simulink model "manul_model_stage15_complete_pre_engineering_20260816"  (R2025a)
settings: Solver=ode3  StartTime=0.0  StopTime=0.3  FixedStep=Ts_power  RelTol=1e-3
InitFcn:
  | run('D:/PV_MPPT/PV_ESS_MPC_Manul_Reproduction/experiments/stage15_bus_stability_20260814/pvess_stage15_busfix_init.m')
values from neighbouring files (symbols this model uses):
  Ad_mpvc = expm(A_mpvc*Ts_mpc)    [pvess_beginner_init_baseline.m]    (also in pvess_stage15_busfix_init.m; pvess_stage15_busfix_init_pre_cpl_20260817.m; pvess_stage15_busfix_init_pre_engineering_20260816.m; pvess_stage15_busfix_init_pre_gridpi_tuning_20260817.m)
  Bd_mpvc = A_mpvc\((Ad_mpvc-eye(2))*B_mpvc)    [pvess_beginner_init_baseline.m]    (also in pvess_stage15_busfix_init.m; pvess_stage15_busfix_init_pre_cpl_20260817.m; pvess_stage15_busfix_init_pre_engineering_20260816.m; pvess_stage15_busfix_init_pre_gridpi_tuning_20260817.m)
  Cdc = 18e-3    (= 0.018)    [pvess_beginner_init_baseline.m]    (also in pvess_stage15_busfix_init.m; pvess_stage15_busfix_init_pre_cpl_20260817.m; pvess_stage15_busfix_init_pre_engineering_20260816.m; pvess_stage15_busfix_init_pre_gridpi_tuning_20260817.m)
  Cpv = 10e-3    (= 0.01)    [pvess_beginner_init_baseline.m]    (also in pvess_stage15_busfix_init.m; pvess_stage15_busfix_init_pre_cpl_20260817.m; pvess_stage15_busfix_init_pre_engineering_20260816.m; pvess_stage15_busfix_init_pre_gridpi_tuning_20260817.m)
  Db0 = 1 - V_bat_nom/Vdc_ref    (= 0.75)    [pvess_beginner_init_baseline.m]    (also in pvess_stage15_busfix_init.m; pvess_stage15_busfix_init_pre_cpl_20260817.m; pvess_stage15_busfix_init_pre_engineering_20260816.m; pvess_stage15_busfix_init_pre_gridpi_tuning_20260817.m)
  Db_max = 0.95    [pvess_beginner_init_baseline.m]    (also in pvess_stage15_busfix_init.m; pvess_stage15_busfix_init_pre_cpl_20260817.m; pvess_stage15_busfix_init_pre_engineering_20260816.m; pvess_stage15_busfix_init_pre_gridpi_tuning_20260817.m)
  Db_min = 0.05    [pvess_beginner_init_baseline.m]    (also in pvess_stage15_busfix_init.m; pvess_stage15_busfix_init_pre_cpl_20260817.m; pvess_stage15_busfix_init_pre_engineering_20260816.m; pvess_stage15_busfix_init_pre_gridpi_tuning_20260817.m)
  Dpv0 = 1 - 547/Vdc_ref    (= 0.544166666667)    [pvess_beginner_init_baseline.m]    (also in pvess_stage15_busfix_init.m; pvess_stage15_busfix_init_pre_cpl_20260817.m; pvess_stage15_busfix_init_pre_engineering_20260816.m; pvess_stage15_busfix_init_pre_gridpi_tuning_20260817.m)
  Dpv_curtail_bias = 0.506    [pvess_stage15_busfix_init.m]    (also in pvess_stage15_busfix_init_pre_cpl_20260817.m; pvess_stage15_busfix_init_pre_engineering_20260816.m; pvess_stage15_busfix_init_pre_gridpi_tuning_20260817.m)
  Dpv_max = 0.75    [pvess_beginner_init_baseline.m]    (also in pvess_stage15_busfix_init.m; pvess_stage15_busfix_init_pre_cpl_20260817.m; pvess_stage15_busfix_init_pre_engineering_20260816.m; pvess_stage15_busfix_init_pre_gridpi_tuning_20260817.m)
  Dpv_min = 0.35    [pvess_beginner_init_baseline.m]    (also in pvess_stage15_busfix_init.m; pvess_stage15_busfix_init_pre_cpl_20260817.m; pvess_stage15_busfix_init_pre_engineering_20260816.m; pvess_stage15_busfix_init_pre_gridpi_tuning_20260817.m)
  Dpv_slew_down = -5.0    (= -5)    [pvess_stage15_busfix_init.m]    (also in pvess_stage15_busfix_init_pre_cpl_20260817.m; pvess_stage15_busfix_init_pre_engineering_20260816.m; pvess_stage15_busfix_init_pre_gridpi_tuning_20260817.m)
  Dpv_slew_up = 1.0    (= 1)    [pvess_stage15_busfix_init.m]    (also in pvess_stage15_busfix_init_pre_cpl_20260817.m; pvess_stage15_busfix_init_pre_engineering_20260816.m; pvess_stage15_busfix_init_pre_gridpi_tuning_20260817.m)
  Dpv_step = 2e-4    (= 0.0002)    [pvess_beginner_init_baseline.m]    (also in pvess_stage15_busfix_init.m; pvess_stage15_busfix_init_pre_cpl_20260817.m; pvess_stage15_busfix_init_pre_engineering_20260816.m; pvess_stage15_busfix_init_pre_gridpi_tuning_20260817.m)
  eps_dI = 1e-3    (= 0.001)    [pvess_beginner_init_baseline.m]    (also in pvess_stage15_busfix_init.m; pvess_stage15_busfix_init_pre_cpl_20260817.m; pvess_stage15_busfix_init_pre_engineering_20260816.m; pvess_stage15_busfix_init_pre_gridpi_tuning_20260817.m)
  eps_dV = 1e-3    (= 0.001)    [pvess_beginner_init_baseline.m]    (also in pvess_stage15_busfix_init.m; pvess_stage15_busfix_init_pre_cpl_20260817.m; pvess_stage15_busfix_init_pre_engineering_20260816.m; pvess_stage15_busfix_init_pre_gridpi_tuning_20260817.m)
  eps_inc = 1e-4    (= 0.0001)    [pvess_beginner_init_baseline.m]    (also in pvess_stage15_busfix_init.m; pvess_stage15_busfix_init_pre_cpl_20260817.m; pvess_stage15_busfix_init_pre_engineering_20260816.m; pvess_stage15_busfix_init_pre_gridpi_tuning_20260817.m)
  f_grid = 50    [pvess_beginner_init_baseline.m]    (also in pvess_stage15_busfix_init.m; pvess_stage15_busfix_init_pre_cpl_20260817.m; pvess_stage15_busfix_init_pre_engineering_20260816.m; pvess_stage15_busfix_init_pre_gridpi_tuning_20260817.m)
  freq_threshold = 0.15    [pvess_beginner_init_baseline.m]    (also in pvess_stage15_busfix_init.m; pvess_stage15_busfix_init_pre_cpl_20260817.m; pvess_stage15_busfix_init_pre_engineering_20260816.m; pvess_stage15_busfix_init_pre_gridpi_tuning_20260817.m)
  Ibat_curtail_release = -0.8*Ibat_max    (= -1333.33333333)    [pvess_stage15_busfix_init.m]    (also in pvess_stage15_busfix_init_pre_cpl_20260817.m; pvess_stage15_busfix_init_pre_engineering_20260816.m; pvess_stage15_busfix_init_pre_gridpi_tuning_20260817.m)
  Ibat_max = P_bat_rated/V_bat_nom    (= 1666.66666667)    [pvess_beginner_init_baseline.m]    (also in pvess_stage15_busfix_init.m; pvess_stage15_busfix_init_pre_cpl_20260817.m; pvess_stage15_busfix_init_pre_engineering_20260816.m; pvess_stage15_busfix_init_pre_gridpi_tuning_20260817.m)
  K_bat_sign = 1    [pvess_beginner_init_baseline.m]    (also in pvess_stage15_busfix_init.m; pvess_stage15_busfix_init_pre_cpl_20260817.m; pvess_stage15_busfix_init_pre_engineering_20260816.m; pvess_stage15_busfix_init_pre_gridpi_tuning_20260817.m)
  K_grid_sign = -1    [pvess_beginner_init_baseline.m]    (also in pvess_stage15_busfix_init.m; pvess_stage15_busfix_init_pre_cpl_20260817.m; pvess_stage15_busfix_init_pre_engineering_20260816.m; pvess_stage15_busfix_init_pre_gridpi_tuning_20260817.m)
  Ki_dc = 3.40748e5    (= 340748)    [pvess_beginner_init_baseline.m]    (also in pvess_stage15_busfix_init.m = 2131834.55064; pvess_stage15_busfix_init_pre_cpl_20260817.m; pvess_stage15_busfix_init_pre_engineering_20260816.m; pvess_stage15_busfix_init_pre_gridpi_tuning_20260817.m)
  Kii_bat = 0.150    (= 0.15)    [pvess_beginner_init_baseline.m]    (also in pvess_stage15_busfix_init.m = 0.05; pvess_stage15_busfix_init_pre_cpl_20260817.m = 0.05; pvess_stage15_busfix_init_pre_engineering_20260816.m = 0.05; pvess_stage15_busfix_init_pre_gridpi_tuning_20260817.m = 0.05)
  Kiv_bat = 650    [pvess_beginner_init_baseline.m]    (also in pvess_stage15_busfix_init.m; pvess_stage15_busfix_init_pre_cpl_20260817.m; pvess_stage15_busfix_init_pre_engineering_20260816.m; pvess_stage15_busfix_init_pre_gridpi_tuning_20260817.m)
  Kp_dc = 3836.125    [pvess_beginner_init_baseline.m]    (also in pvess_stage15_busfix_init.m = 2*zeta_dc*(2*pi*f_bw_dc)*Cdc*Vdc_ref; pvess_stage15_busfix_init_pre_cpl_20260817.m; pvess_stage15_busfix_init_pre_engineering_20260816.m; pvess_stage15_busfix_init_pre_gridpi_tuning_20260817.m)
  Kp_pv_curtail = 5e-5    (= 5e-05)    [pvess_stage15_busfix_init.m]    (also in pvess_stage15_busfix_init_pre_cpl_20260817.m; pvess_stage15_busfix_init_pre_engineering_20260816.m; pvess_stage15_busfix_init_pre_gridpi_tuning_20260817.m)
  Kpi_bat = 100e-3    (= 0.1)    [pvess_beginner_init_baseline.m]    (also in pvess_stage15_busfix_init.m = 0.005; pvess_stage15_busfix_init_pre_cpl_20260817.m = 0.005; pvess_stage15_busfix_init_pre_engineering_20260816.m = 0.005; pvess_stage15_busfix_init_pre_gridpi_tuning_20260817.m = 0.005)
  Kpv_bat = 4    [pvess_beginner_init_baseline.m]    (also in pvess_stage15_busfix_init.m; pvess_stage15_busfix_init_pre_cpl_20260817.m; pvess_stage15_busfix_init_pre_engineering_20260816.m; pvess_stage15_busfix_init_pre_gridpi_tuning_20260817.m)
  lambda_mppc = 0.001    [pvess_beginner_init_baseline.m]    (also in pvess_stage15_busfix_init.m; pvess_stage15_busfix_init_pre_cpl_20260817.m; pvess_stage15_busfix_init_pre_engineering_20260816.m; pvess_stage15_busfix_init_pre_gridpi_tuning_20260817.m)
  lambda_mpvc = 3e-6    (= 3e-06)    [pvess_beginner_init_baseline.m]    (also in pvess_stage15_busfix_init.m; pvess_stage15_busfix_init_pre_cpl_20260817.m; pvess_stage15_busfix_init_pre_engineering_20260816.m; pvess_stage15_busfix_init_pre_gridpi_tuning_20260817.m)
  Lbat = 11.25e-3    (= 0.01125)    [pvess_beginner_init_baseline.m]    (also in pvess_stage15_busfix_init.m = 0.0005; pvess_stage15_busfix_init_pre_cpl_20260817.m = 0.0005; pvess_stage15_busfix_init_pre_engineering_20260816.m = 0.0005; pvess_stage15_busfix_init_pre_gridpi_tuning_20260817.m = 0.0005)
  Lf = 0.6e-3    (= 0.0006)    [pvess_beginner_init_baseline.m]    (also in pvess_stage15_busfix_init.m; pvess_stage15_busfix_init_pre_cpl_20260817.m; pvess_stage15_busfix_init_pre_engineering_20260816.m; pvess_stage15_busfix_init_pre_gridpi_tuning_20260817.m)
  Lpv = 0.8e-3    (= 0.0008)    [pvess_beginner_init_baseline.m]    (also in pvess_stage15_busfix_init.m; pvess_stage15_busfix_init_pre_cpl_20260817.m; pvess_stage15_busfix_init_pre_engineering_20260816.m; pvess_stage15_busfix_init_pre_gridpi_tuning_20260817.m)
  m_var = 4e6    (= 4000000)    [pvess_beginner_init_baseline.m]    (also in pvess_stage15_busfix_init.m; pvess_stage15_busfix_init_pre_cpl_20260817.m; pvess_stage15_busfix_init_pre_engineering_20260816.m; pvess_stage15_busfix_init_pre_gridpi_tuning_20260817.m)
  N_ems_fast_avg = 100    [pvess_beginner_init_baseline.m]    (also in pvess_stage15_busfix_init.m; pvess_stage15_busfix_init_pre_cpl_20260817.m; pvess_stage15_busfix_init_pre_engineering_20260816.m; pvess_stage15_busfix_init_pre_gridpi_tuning_20260817.m)
  omega_grid = 2*pi*f_grid    (= 314.159265359)    [pvess_beginner_init_baseline.m]    (also in pvess_stage15_busfix_init.m; pvess_stage15_busfix_init_pre_cpl_20260817.m; pvess_stage15_busfix_init_pre_engineering_20260816.m; pvess_stage15_busfix_init_pre_gridpi_tuning_20260817.m)
  P_base_mpc = 2e6    (= 2000000)    [pvess_beginner_init_baseline.m]    (also in pvess_stage15_busfix_init.m; pvess_stage15_busfix_init_pre_cpl_20260817.m; pvess_stage15_busfix_init_pre_engineering_20260816.m; pvess_stage15_busfix_init_pre_gridpi_tuning_20260817.m)
  phase_threshold = 0.99863    [pvess_beginner_init_baseline.m]    (also in pvess_stage15_busfix_init.m; pvess_stage15_busfix_init_pre_cpl_20260817.m; pvess_stage15_busfix_init_pre_engineering_20260816.m; pvess_stage15_busfix_init_pre_gridpi_tuning_20260817.m)
  Pref_max = 2.2e6    (= 2200000)    [pvess_beginner_init_baseline.m]    (also in pvess_stage15_busfix_init.m; pvess_stage15_busfix_init_pre_cpl_20260817.m; pvess_stage15_busfix_init_pre_engineering_20260816.m; pvess_stage15_busfix_init_pre_gridpi_tuning_20260817.m)
  Pref_min = -2.2e6    (= -2200000)    [pvess_beginner_init_baseline.m]    (also in pvess_stage15_busfix_init.m; pvess_stage15_busfix_init_pre_cpl_20260817.m; pvess_stage15_busfix_init_pre_engineering_20260816.m; pvess_stage15_busfix_init_pre_gridpi_tuning_20260817.m)
  Q_base_mpc = 1e6    (= 1000000)    [pvess_beginner_init_baseline.m]    (also in pvess_stage15_busfix_init.m; pvess_stage15_busfix_init_pre_cpl_20260817.m; pvess_stage15_busfix_init_pre_engineering_20260816.m; pvess_stage15_busfix_init_pre_gridpi_tuning_20260817.m)
  Q_bat_Ah = 1300    [pvess_beginner_init_baseline.m]    (also in pvess_stage15_busfix_init.m; pvess_stage15_busfix_init_pre_cpl_20260817.m; pvess_stage15_busfix_init_pre_engineering_20260816.m; pvess_stage15_busfix_init_pre_gridpi_tuning_20260817.m)
  R_bat_internal = 0.02    [pvess_beginner_init_baseline.m]    (also in pvess_stage15_busfix_init.m; pvess_stage15_busfix_init_pre_cpl_20260817.m; pvess_stage15_busfix_init_pre_engineering_20260816.m; pvess_stage15_busfix_init_pre_gridpi_tuning_20260817.m)
  Rf = 0.019    [pvess_beginner_init_baseline.m]    (also in pvess_stage15_busfix_init.m; pvess_stage15_busfix_init_pre_cpl_20260817.m; pvess_stage15_busfix_init_pre_engineering_20260816.m; pvess_stage15_busfix_init_pre_gridpi_tuning_20260817.m)
  RLbat = 2e-3    (= 0.002)    [pvess_beginner_init_baseline.m]    (also in pvess_stage15_busfix_init.m; pvess_stage15_busfix_init_pre_cpl_20260817.m; pvess_stage15_busfix_init_pre_engineering_20260816.m; pvess_stage15_busfix_init_pre_gridpi_tuning_20260817.m)
  RLpv = 2e-3    (= 0.002)    [pvess_beginner_init_baseline.m]    (also in pvess_stage15_busfix_init.m; pvess_stage15_busfix_init_pre_cpl_20260817.m; pvess_stage15_busfix_init_pre_engineering_20260816.m; pvess_stage15_busfix_init_pre_gridpi_tuning_20260817.m)
  S_tr = 2.5e6    (= 2500000)    [pvess_beginner_init_baseline.m]    (also in pvess_stage15_busfix_init.m; pvess_stage15_busfix_init_pre_cpl_20260817.m; pvess_stage15_busfix_init_pre_engineering_20260816.m; pvess_stage15_busfix_init_pre_gridpi_tuning_20260817.m)
  SOC0 = 50    [pvess_beginner_init_baseline.m]    (also in pvess_stage15_busfix_init.m; pvess_stage15_busfix_init_pre_cpl_20260817.m; pvess_stage15_busfix_init_pre_engineering_20260816.m; pvess_stage15_busfix_init_pre_gridpi_tuning_20260817.m)
  SOC_max = 90    [pvess_beginner_init_baseline.m]    (also in pvess_stage15_busfix_init.m; pvess_stage15_busfix_init_pre_cpl_20260817.m; pvess_stage15_busfix_init_pre_engineering_20260816.m; pvess_stage15_busfix_init_pre_gridpi_tuning_20260817.m)
  SOC_min = 10    [pvess_beginner_init_baseline.m]    (also in pvess_stage15_busfix_init.m; pvess_stage15_busfix_init_pre_cpl_20260817.m; pvess_stage15_busfix_init_pre_engineering_20260816.m; pvess_stage15_busfix_init_pre_gridpi_tuning_20260817.m)
  sync_hold = 0.1    [pvess_beginner_init_baseline.m]    (also in pvess_stage15_busfix_init.m; pvess_stage15_busfix_init_pre_cpl_20260817.m; pvess_stage15_busfix_init_pre_engineering_20260816.m; pvess_stage15_busfix_init_pre_gridpi_tuning_20260817.m)
  T_ac_step = 0.2    [pvess_beginner_init_baseline.m]    (also in pvess_stage15_busfix_init.m = 0.5; pvess_stage15_busfix_init_pre_cpl_20260817.m = 0.5; pvess_stage15_busfix_init_pre_engineering_20260816.m = 0.5; pvess_stage15_busfix_init_pre_gridpi_tuning_20260817.m = 0.5)
  T_grid_connect = 1.6    [pvess_beginner_init_baseline.m]    (also in pvess_stage15_busfix_init.m; pvess_stage15_busfix_init_pre_cpl_20260817.m; pvess_stage15_busfix_init_pre_engineering_20260816.m; pvess_stage15_busfix_init_pre_gridpi_tuning_20260817.m)
  T_grid_dip = 3.5    [pvess_beginner_init_baseline.m]    (also in pvess_stage15_busfix_init.m; pvess_stage15_busfix_init_pre_cpl_20260817.m; pvess_stage15_busfix_init_pre_engineering_20260816.m; pvess_stage15_busfix_init_pre_gridpi_tuning_20260817.m)
  T_sync = 1.4    [pvess_beginner_init_baseline.m]    (also in pvess_stage15_busfix_init.m; pvess_stage15_busfix_init_pre_cpl_20260817.m; pvess_stage15_busfix_init_pre_engineering_20260816.m; pvess_stage15_busfix_init_pre_gridpi_tuning_20260817.m)
  Ts_bat_ctrl = 100e-6    (= 0.0001)    [pvess_beginner_init_baseline.m]    (also in pvess_stage15_busfix_init.m; pvess_stage15_busfix_init_pre_cpl_20260817.m; pvess_stage15_busfix_init_pre_engineering_20260816.m; pvess_stage15_busfix_init_pre_gridpi_tuning_20260817.m)
  Ts_ems = 1e-3    (= 0.001)    [pvess_beginner_init_baseline.m]    (also in pvess_stage15_busfix_init.m; pvess_stage15_busfix_init_pre_cpl_20260817.m; pvess_stage15_busfix_init_pre_engineering_20260816.m; pvess_stage15_busfix_init_pre_gridpi_tuning_20260817.m)
  Ts_mpc = 1/20e3    (= 5e-05)    [pvess_beginner_init_baseline.m]    (also in pvess_stage15_busfix_init.m; pvess_stage15_busfix_init_pre_cpl_20260817.m; pvess_stage15_busfix_init_pre_engineering_20260816.m; pvess_stage15_busfix_init_pre_gridpi_tuning_20260817.m)
  Ts_mppt = 1e-3    (= 0.001)    [pvess_beginner_init_baseline.m]    (also in pvess_stage15_busfix_init.m; pvess_stage15_busfix_init_pre_cpl_20260817.m; pvess_stage15_busfix_init_pre_engineering_20260816.m; pvess_stage15_busfix_init_pre_gridpi_tuning_20260817.m)
  Ts_power = 2e-6    (= 2e-06)    [pvess_beginner_init_baseline.m]    (also in pvess_stage15_busfix_init.m; pvess_stage15_busfix_init_pre_cpl_20260817.m; pvess_stage15_busfix_init_pre_engineering_20260816.m; pvess_stage15_busfix_init_pre_gridpi_tuning_20260817.m)
  Ts_soc = 1e-4    (= 0.0001)    [pvess_beginner_init_baseline.m]    (also in pvess_stage15_busfix_init.m; pvess_stage15_busfix_init_pre_cpl_20260817.m; pvess_stage15_busfix_init_pre_engineering_20260816.m; pvess_stage15_busfix_init_pre_gridpi_tuning_20260817.m)
  V_bat_nom = 300    [pvess_beginner_init_baseline.m]    (also in pvess_stage15_busfix_init.m; pvess_stage15_busfix_init_pre_cpl_20260817.m; pvess_stage15_busfix_init_pre_engineering_20260816.m; pvess_stage15_busfix_init_pre_gridpi_tuning_20260817.m)
  V_tr_hv = 25e3    (= 25000)    [pvess_beginner_init_baseline.m]    (also in pvess_stage15_busfix_init.m; pvess_stage15_busfix_init_pre_cpl_20260817.m; pvess_stage15_busfix_init_pre_engineering_20260816.m; pvess_stage15_busfix_init_pre_gridpi_tuning_20260817.m)
  V_tr_lv = Vac_ll    (= 690)    [pvess_beginner_init_baseline.m]    (also in pvess_stage15_busfix_init.m; pvess_stage15_busfix_init_pre_cpl_20260817.m; pvess_stage15_busfix_init_pre_engineering_20260816.m; pvess_stage15_busfix_init_pre_gridpi_tuning_20260817.m)
  Vac_phase_peak = sqrt(2)*Vac_ll/sqrt(3)    [pvess_beginner_init_baseline.m]    (also in pvess_stage15_busfix_init.m; pvess_stage15_busfix_init_pre_cpl_20260817.m; pvess_stage15_busfix_init_pre_engineering_20260816.m; pvess_stage15_busfix_init_pre_gridpi_tuning_20260817.m)
  Vdc_curtail_off = 1185    [pvess_stage15_busfix_init.m]    (also in pvess_stage15_busfix_init_pre_cpl_20260817.m; pvess_stage15_busfix_init_pre_engineering_20260816.m; pvess_stage15_busfix_init_pre_gridpi_tuning_20260817.m)
  Vdc_curtail_on = 1220    [pvess_stage15_busfix_init.m]    (also in pvess_stage15_busfix_init_pre_cpl_20260817.m; pvess_stage15_busfix_init_pre_engineering_20260816.m; pvess_stage15_busfix_init_pre_gridpi_tuning_20260817.m)
  Vdc_ref = 1200    [pvess_beginner_init_baseline.m]    (also in pvess_stage15_busfix_init.m; pvess_stage15_busfix_init_pre_cpl_20260817.m; pvess_stage15_busfix_init_pre_engineering_20260816.m; pvess_stage15_busfix_init_pre_gridpi_tuning_20260817.m)
  Vf_diode = 1.0    (= 1)    [pvess_beginner_init_baseline.m]    (also in pvess_stage15_busfix_init.m; pvess_stage15_busfix_init_pre_cpl_20260817.m; pvess_stage15_busfix_init_pre_engineering_20260816.m; pvess_stage15_busfix_init_pre_gridpi_tuning_20260817.m)
  Vpv0 = 547    [pvess_beginner_init_baseline.m]    (also in pvess_stage15_busfix_init.m; pvess_stage15_busfix_init_pre_cpl_20260817.m; pvess_stage15_busfix_init_pre_engineering_20260816.m; pvess_stage15_busfix_init_pre_gridpi_tuning_20260817.m)
  Vsync_threshold = 10    [pvess_beginner_init_baseline.m]    (also in pvess_stage15_busfix_init.m; pvess_stage15_busfix_init_pre_cpl_20260817.m; pvess_stage15_busfix_init_pre_engineering_20260816.m; pvess_stage15_busfix_init_pre_gridpi_tuning_20260817.m)
undefined symbols (not defined in the file or in its folder): DiscIntNeverNeededParam, dspblkCoreblockFVToolHelper, gcbh, Ion, Kt_dc, Lithium
libraries: dspstat3 x10, simulink x9, spsBreakerLib x5, spsCurrentMeasurementLib x4, slpidlib x3, spsThreePhaseVIMeasurementLib x3, eeRmsMeasurement x3, spsThreePhaseParallelRLCLoadLib x3, spsThreePhaseBreakerLib x3, spsParallelRLCBranchLib x2, spsVariableResistorLib x2, spsThreePhaseSeriesRLCBranchLib x2
(part 2 of 2)

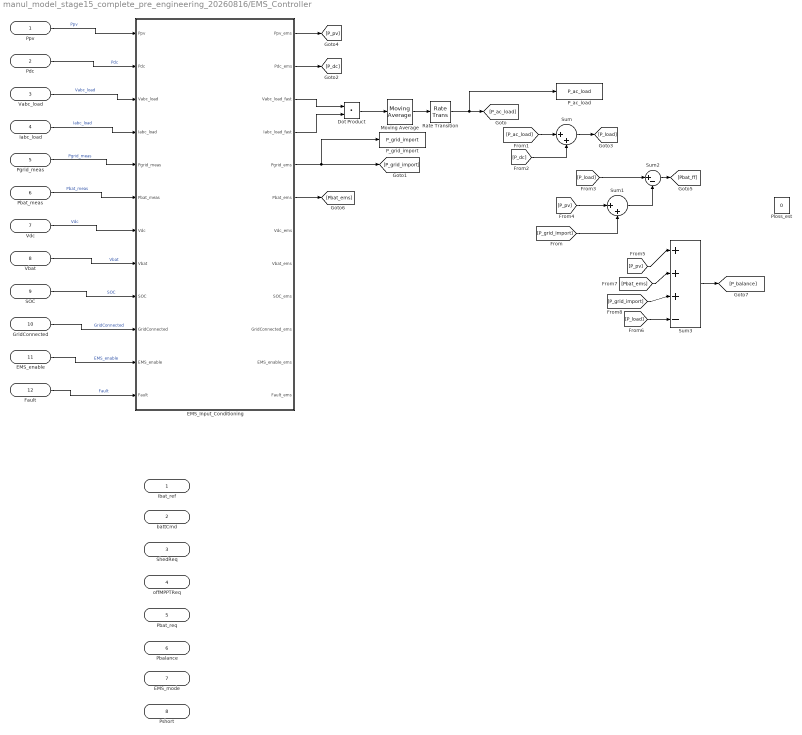
== system manul_model_stage15_complete_pre_engineering_20260816/EMS_Controller ==
  Ppv : Inport  OutDataTypeStr=double  PortDimensions=1  SampleTime=Ts_power
  Pdc : Inport  Port=2  OutDataTypeStr=double  PortDimensions=1  SampleTime=Ts_power
  Vabc_load : Inport  Port=3  OutDataTypeStr=double  PortDimensions=3  SampleTime=Ts_mpc
  Iabc_load : Inport  Port=4  OutDataTypeStr=double  PortDimensions=3  SampleTime=Ts_mpc
  Pgrid_meas : Inport  Port=5  OutDataTypeStr=double  PortDimensions=1  SampleTime=Ts_mpc
  Pbat_meas : Inport  Port=6  OutDataTypeStr=double  PortDimensions=1  SampleTime=Ts_power
  Vdc : Inport  Port=7  OutDataTypeStr=double  PortDimensions=1  SampleTime=Ts_power
  Vbat : Inport  Port=8  OutDataTypeStr=double  PortDimensions=1  SampleTime=Ts_power
  SOC : Inport  Port=9  OutDataTypeStr=double  PortDimensions=1  SampleTime=Ts_soc
  GridConnected : Inport  Port=10  OutDataTypeStr=boolean  PortDimensions=1
  EMS_enable : Inport  Port=11  OutDataTypeStr=boolean  PortDimensions=1
  Fault : Inport  Port=12  OutDataTypeStr=boolean  PortDimensions=1
  Dot Product : DotProduct  OutDataTypeStr=Inherit: Inherit via internal rule
  EMS_Input_Conditioning : Subsystem
  Moving Average : dspstat3/Moving Average  Method=Sliding window  ForgettingFactorPort=off  SpecifyWindowLength=on  WindowLength=20  OverlapLength=19  AllowArbitraryInputLength=off  ForgettingFactor=0.9  SimulateUsing=Interpreted execution
  P_ac_load : ToWorkspace  VariableName=P_ac_load  SaveFormat=Timeseries  SampleTime=-1
  P_grid_import : ToWorkspace  VariableName=P_grid_import  SaveFormat=Timeseries  SampleTime=-1
  Ploss_est : Constant  Value=0
  Rate Transition : RateTransition  OutPortSampleTime=Ts_ems
  Sum : Sum  Inputs=|++
  Sum1 : Sum  Inputs=|++
  Sum2 : Sum  Inputs=|+-
  Sum3 : Sum  Inputs=|+++-
  Ibat_ref : Outport  OutDataTypeStr=double  PortDimensions=1
  battCmd : Outport  Port=2  OutDataTypeStr=int8  PortDimensions=1
  ShedReq : Outport  Port=3  OutDataTypeStr=boolean  PortDimensions=1
  offMPPTReq : Outport  Port=4  OutDataTypeStr=boolean  PortDimensions=1
  Pbat_req : Outport  Port=5  OutDataTypeStr=double  PortDimensions=1
  Pbalance : Outport  Port=6  OutDataTypeStr=double  PortDimensions=1
  EMS_mode : Outport  Port=7  OutDataTypeStr=int8  PortDimensions=1
  Pshort : Outport  Port=8  OutDataTypeStr=double  PortDimensions=1
  wires:
  Ppv/1 -> EMS_Input_Conditioning/1(Ppv)  "Ppv"
  Pdc/1 -> EMS_Input_Conditioning/2(Pdc)  "Pdc"
  Vabc_load/1 -> EMS_Input_Conditioning/3(Vabc_load)  "Vabc_load"
  Iabc_load/1 -> EMS_Input_Conditioning/4(Iabc_load)  "Iabc_load"
  Pgrid_meas/1 -> EMS_Input_Conditioning/5(Pgrid_meas)  "Pgrid_meas"
  Pbat_meas/1 -> EMS_Input_Conditioning/6(Pbat_meas)  "Pbat_meas"
  Vdc/1 -> EMS_Input_Conditioning/7(Vdc)  "Vdc"
  Vbat/1 -> EMS_Input_Conditioning/8(Vbat)  "Vbat"
  SOC/1 -> EMS_Input_Conditioning/9(SOC)  "SOC"
  GridConnected/1 -> EMS_Input_Conditioning/10(GridConnected)  "GridConnected"
  EMS_enable/1 -> EMS_Input_Conditioning/11(EMS_enable)  "EMS_enable"
  Fault/1 -> EMS_Input_Conditioning/12(Fault)  "Fault"
  EMS_Input_Conditioning/3(Vabc_load_fast) -> Dot Product/1
  EMS_Input_Conditioning/4(Iabc_load_fast) -> Dot Product/2
  Dot Product/1 -> Moving Average/1
  Moving Average/1 -> Rate Transition/1
  Rate Transition/1 -> P_ac_load/1, [P_ac_load]
  EMS_Input_Conditioning/5(Pgrid_ems) -> P_grid_import/1, [P_grid_import]
  EMS_Input_Conditioning/2(Pdc_ems) -> [P_dc]
  [P_ac_load] -> Sum/1
  [P_dc] -> Sum/2
  Sum/1 -> [P_load]
  EMS_Input_Conditioning/1(Ppv_ems) -> [P_pv]
  [P_pv] -> Sum1/1
  [P_grid_import] -> Sum1/2
  Sum2/1 -> [Pbat_ff]
  [P_load] -> Sum2/1
  Sum1/1 -> Sum2/2
  [P_pv] -> Sum3/1
  [P_load] -> Sum3/4
  EMS_Input_Conditioning/6(Pbat_ems) -> [Pbat_ems]
  [Pbat_ems] -> Sum3/2
  [P_grid_import] -> Sum3/3
  Sum3/1 -> [P_balance]

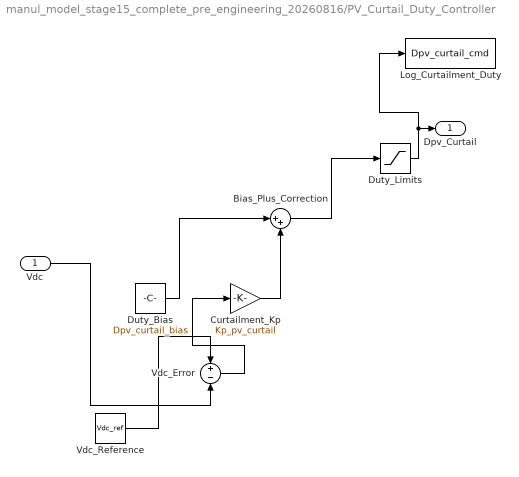
== system manul_model_stage15_complete_pre_engineering_20260816/PV_Curtail_Duty_Controller ==
  Vdc : Inport
  Bias_Plus_Correction : Sum  Inputs=|++
  Curtailment_Kp : Gain  Gain=Kp_pv_curtail
  Duty_Bias : Constant  Value=Dpv_curtail_bias
  Duty_Limits : Saturate  UpperLimit=Dpv_max  LowerLimit=Dpv_min
  Log_Curtailment_Duty : ToWorkspace  VariableName=Dpv_curtail_cmd  SaveFormat=Timeseries
      settings: Decimation=20
  Vdc_Error : Sum  Inputs=+-
  Vdc_Reference : Constant  Value=Vdc_ref
  Dpv_Curtail : Outport
  wires:
  Vdc_Reference/1 -> Vdc_Error/1
  Vdc/1 -> Vdc_Error/2
  Vdc_Error/1 -> Curtailment_Kp/1
  Curtailment_Kp/1 -> Bias_Plus_Correction/2
  Duty_Bias/1 -> Bias_Plus_Correction/1
  Bias_Plus_Correction/1 -> Duty_Limits/1
  Duty_Limits/1 -> Log_Curtailment_Duty/1, Dpv_Curtail/1

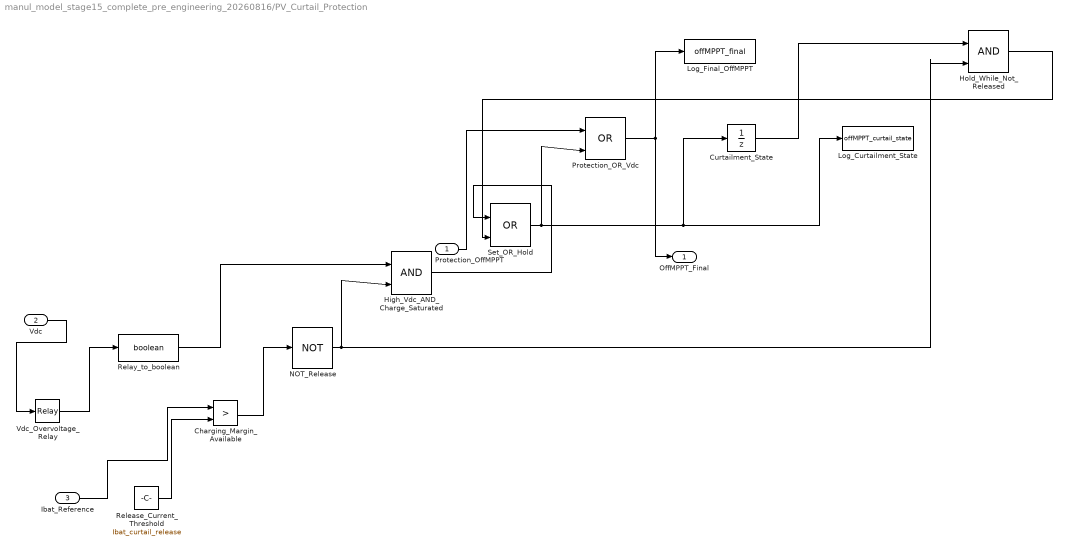
== system manul_model_stage15_complete_pre_engineering_20260816/PV_Curtail_Protection ==
  Protection_OffMPPT : Inport
  Vdc : Inport  Port=2
  Ibat_Reference : Inport  Port=3
  Charging_Margin_Available : RelationalOperator  Operator=>
  Curtailment_State : UnitDelay  SampleTime=Ts_bat_ctrl
  High_Vdc_AND_Charge_Saturated : Logic  IconShape=distinctive
  Hold_While_Not_Released : Logic  IconShape=distinctive
  Log_Curtailment_State : ToWorkspace  VariableName=offMPPT_curtail_state  SaveFormat=Timeseries
      settings: Decimation=20
  Log_Final_OffMPPT : ToWorkspace  VariableName=offMPPT_final  SaveFormat=Timeseries
      settings: Decimation=20
  NOT_Release : Logic  Operator=NOT  Inputs=1  IconShape=distinctive
  Protection_OR_Vdc : Logic  Operator=OR  IconShape=distinctive
  Relay_to_boolean : DataTypeConversion  OutDataTypeStr=boolean
  Release_Current_Threshold : Constant  Value=Ibat_curtail_release
  Set_OR_Hold : Logic  Operator=OR  IconShape=distinctive
  Vdc_Overvoltage_Relay : Relay  OnSwitchValue=Vdc_curtail_on  OffSwitchValue=Vdc_curtail_off  OutDataTypeStr=double
  OffMPPT_Final : Outport
  wires:
  Ibat_Reference/1 -> Charging_Margin_Available/1
  Release_Current_Threshold/1 -> Charging_Margin_Available/2
  Charging_Margin_Available/1 -> NOT_Release/1
  NOT_Release/1 -> High_Vdc_AND_Charge_Saturated/2, Hold_While_Not_Released/2
  Curtailment_State/1 -> Hold_While_Not_Released/1
  Hold_While_Not_Released/1 -> Set_OR_Hold/2
  High_Vdc_AND_Charge_Saturated/1 -> Set_OR_Hold/1
  Set_OR_Hold/1 -> Log_Curtailment_State/1, Curtailment_State/1, Protection_OR_Vdc/2
  Relay_to_boolean/1 -> High_Vdc_AND_Charge_Saturated/1
  Protection_OffMPPT/1 -> Protection_OR_Vdc/1
  Vdc/1 -> Vdc_Overvoltage_Relay/1
  Vdc_Overvoltage_Relay/1 -> Relay_to_boolean/1
  Protection_OR_Vdc/1 -> OffMPPT_Final/1, Log_Final_OffMPPT/1

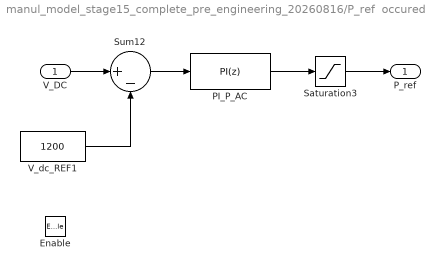
== system manul_model_stage15_complete_pre_engineering_20260816/P_ref  occured ==
  V_DC : Inport
  Enable : EnablePort
  PI_P_AC : slpidlib/PID Controller  Controller=PI  Form=Parallel  TimeDomain=Discrete-time  UseExternalTs=off  SampleTime=Ts_mpc  IntegratorMethod=Forward Euler  FilterMethod=Forward Euler  ControllerParametersSource=internal  P=Kp_dc  I=Ki_dc  UseKiTs=off  D=0  UseExternalDerivativeSource=off  N=100  UseFilter=on  TunerSelectOption=Transfer Function Based (PID Tuner App)  InitialConditionSource=internal  InitialConditionForIntegrator=0  InitialConditionForFilter=0  DifferentiatorICPrevScaledInput=0  ExternalReset=none  TrackingMode=off  Kt=Kt_dc  LimitOutput=on  SatLimitsSource=internal  UpperSaturationLimit=Pref_max  LowerSaturationLimit=Pref_min  LinearizeAsGain=off  AntiWindupMode=clamping  Kb=1  LimitIntegrator=off  UpperIntegratorSaturationLimit=inf  LowerIntegratorSaturationLimit=-inf  POutMin=[]  POutMax=[]  IOutMin=[]  IOutMax=[]  DOutMin=[]  DOutMax=[]  NOutMin=[]  NOutMax=[]  SumOutMin=[]  SumOutMax=[]  SaturationOutMin=[]  SaturationOutMax=[]  PParamMin=[]  PParamMax=[]  IParamMin=[]  IParamMax=[]  DParamMin=[]  DParamMax=[]  NParamMin=[]  NParamMax=[]  KbParamMin=[]  KbParamMax=[]  KtParamMin=[]  KtParamMax=[]  KbOutMin=[]  KbOutMax=[]  KtOutMin=[]  KtOutMax=[]  IntegratorOutMin=[]  IntegratorOutMax=[]  FilterOutMin=[]  FilterOutMax=[]  SumI1OutMin=[]  SumI1OutMax=[]  SumI2OutMin=[]  SumI2OutMax=[]  SumI3OutMin=[]  SumI3OutMax=[]  SumI4OutMin=[]  SumI4OutMax=[]  SumDOutMin=[]  SumDOutMax=[]  DifferentiatorOutMin=[]  DifferentiatorOutMax=[]  FilterDiffOutCoefMin=[]  FilterDiffOutCoefMax=[]  ReciprocalOutMin=[]  ReciprocalOutMax=[]  SumDenOutMin=[]  SumDenOutMax=[]  SumNumOutMin=[]  SumNumOutMax=[]  DivideOutMin=[]  DivideOutMax=[]  UdiffTsProdOutMin=[]  UdiffTsProdOutMax=[]  NTsProdOutMin=[]  NTsProdOutMax=[]  UintegralTsProdOutMin=[]  UintegralTsProdOutMax=[]  UngainTsProdOutMin=[]  UngainTsProdOutMax=[]  ClampingZeroOutDataTypeStr=Inherit: Inherit via back propagation  ClampingZeroOutMin=[]  ClampingZeroOutMax=[]  FilterDenConstantOutDataTypeStr=Inherit: Inherit via back propagation  FilterDenConstantOutMin=[]  FilterDenConstantOutMax=[]  PCopyOutDataTypeStr=Inherit: Inherit via back propagation  PCopyOutMin=[]  PCopyOutMax=[]  NCopyOutDataTypeStr=Inherit: Inherit via back propagation  NCopyOutMin=[]  NCopyOutMax=[]  IntegratorContinuousStateAttributes=''  IntegratorStateMustResolveToSignalObject=off  IntegratorRTWStateStorageClass=Auto  FilterContinuousStateAttributes=''  FilterStateMustResolveToSignalObject=off  FilterRTWStateStorageClass=Auto  ParallelPVariant=InternalParameters  IdealPVariant=Disabled  IVariant=InternalParameters  DVariant=Disabled  IntegratorVariant=Discrete  SatVariant=Enabled  AWVariant=DiscClampingParallel  PCopyVariant=Disabled  TRVariant=Disabled  FdbkBlocksVariant=Forward  IdealPFdbkVariant=Disabled  SatFdbkVariant=Disabled  DerivativeFilterVariant=Disabled  NVariant=Disabled  NCopyVariant=Disabled_SignalSpec  FilterICVariant=Disabled  IntegratorICVariant=InternalICs  ExternalResetVariant=Disabled  TRSumVariant=Passthrough  SumFdbkVariant=Disabled  SumVariant=Sum_PI  TsampFilterVariant=InternalTs  TsampNgainVariant=Passthrough  TsampIntegralVariant=Disabled_SignalSpec  ExternalSaturationOutDataTypeStr=Inherit: Same as second input  DerivativeSourceVariant=Disabled  PreIntVariant=InternalPreInt
      settings: LibrarySourceBlock=simulink/Discrete/Discrete PID Controller
  Saturation3 : Saturate  UpperLimit=Pref_max  LowerLimit=Pref_min
  Sum12 : Sum  Inputs=|+-
  V_dc_REF1 : Constant  Value=1200
  P_ref : Outport
  wires:
  Sum12/1 -> PI_P_AC/1
  PI_P_AC/1 -> Saturation3/1
  Saturation3/1 -> P_ref/1
  V_DC/1 -> Sum12/1
  V_dc_REF1/1 -> Sum12/2

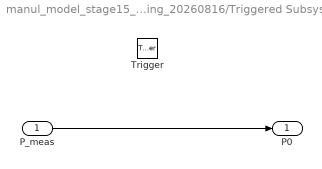
== system manul_model_stage15_complete_pre_engineering_20260816/Triggered Subsystem ==
  P_meas : Inport
  Trigger : TriggerPort  VariantControl=(inherit)
  P0 : Outport
  wires:
  P_meas/1 -> P0/1

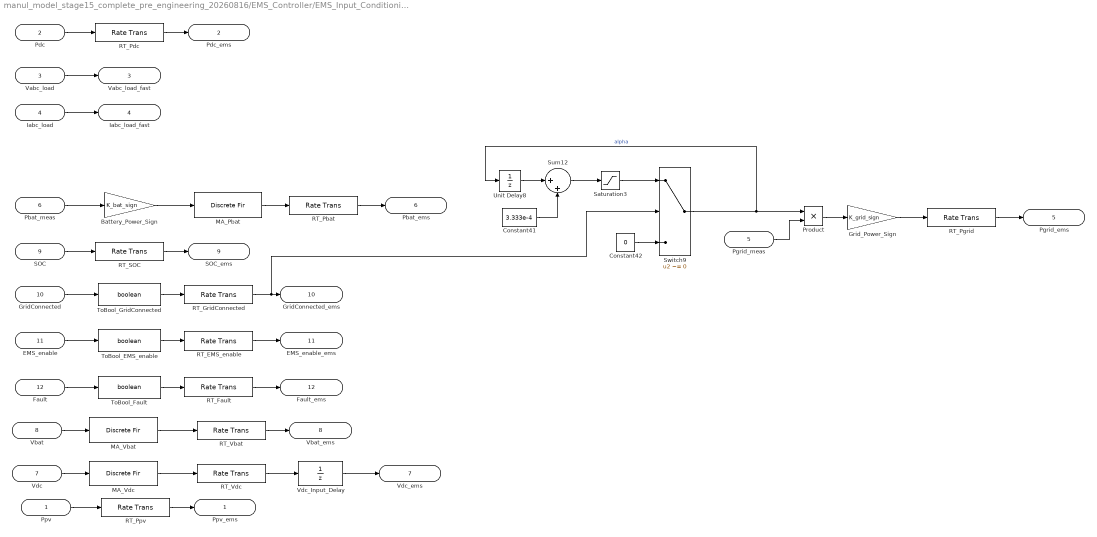
== system manul_model_stage15_complete_pre_engineering_20260816/EMS_Controller/EMS_Input_Conditioning ==
  Ppv : Inport  OutDataTypeStr=double  PortDimensions=1
  Pdc : Inport  Port=2  OutDataTypeStr=double  PortDimensions=1
  Vabc_load : Inport  Port=3  OutDataTypeStr=double  PortDimensions=3
  Iabc_load : Inport  Port=4  OutDataTypeStr=double  PortDimensions=3
  Pgrid_meas : Inport  Port=5  OutDataTypeStr=double  PortDimensions=1
  Pbat_meas : Inport  Port=6  OutDataTypeStr=double  PortDimensions=1
  Vdc : Inport  Port=7  OutDataTypeStr=double  PortDimensions=1
  Vbat : Inport  Port=8  OutDataTypeStr=double  PortDimensions=1
  SOC : Inport  Port=9  OutDataTypeStr=double  PortDimensions=1
  GridConnected : Inport  Port=10  OutDataTypeStr=boolean  PortDimensions=1
  EMS_enable : Inport  Port=11  OutDataTypeStr=boolean  PortDimensions=1
  Fault : Inport  Port=12  OutDataTypeStr=boolean  PortDimensions=1
  Battery_Power_Sign : Gain  Gain=K_bat_sign
  Constant41 : Constant  Value=3.333e-4
  Constant42 : Constant  Value=0
  Grid_Power_Sign : Gain  Gain=K_grid_sign
  MA_Pbat : DiscreteFir  LoadFcn=dspblkCoreblockFVToolHelper(gcbh,'load');  Coefficients=ones(1,N_ems_fast_avg)/N_ems_fast_avg  SampleTime=Ts_power
      settings: CopyFcn=dspblkCoreblockFVToolHelper(gcbh,'copy');  DeleteFcn=dspblkCoreblockFVToolHelper(gcbh,'close');  ModelCloseFcn=dspblkCoreblockFVToolHelper(gcbh,'close');  PreSaveFcn=dspblkCoreblockFVToolHelper(gcbh,'presave');  PostSaveFcn=dspblkCoreblockFVToolHelper(gcbh,'postsave');  CloseFcn=dspblkCoreblockFVToolHelper(gcbh,'close');
  MA_Vbat : DiscreteFir  Coefficients=ones(1,N_ems_fast_avg)/N_ems_fast_avg  InitialStates=V_bat_nom  SampleTime=Ts_power
  MA_Vdc : DiscreteFir  Coefficients=ones(1,N_ems_fast_avg)/N_ems_fast_avg  InitialStates=Vdc_ref  SampleTime=Ts_power
  Product : Product
  RT_EMS_enable : RateTransition  OutPortSampleTime=Ts_ems
  RT_Fault : RateTransition  OutPortSampleTime=Ts_ems
  RT_GridConnected : RateTransition  OutPortSampleTime=Ts_ems
  RT_Pbat : RateTransition  OutPortSampleTime=Ts_ems
  RT_Pdc : RateTransition  OutPortSampleTime=Ts_ems
  RT_Pgrid : RateTransition  OutPortSampleTime=Ts_ems
  RT_Ppv : RateTransition  OutPortSampleTime=Ts_ems
  RT_SOC : RateTransition  OutPortSampleTime=Ts_ems
  RT_Vbat : RateTransition  OutPortSampleTime=Ts_ems
  RT_Vdc : RateTransition  OutPortSampleTime=Ts_ems
  Saturation3 : Saturate  UpperLimit=1  LowerLimit=0
  Sum12 : Sum  Inputs=|++
  Switch9 : Switch  Criteria=u2 ~= 0  SaturateOnIntegerOverflow=off  InputSameDT=off
  ToBool_EMS_enable : DataTypeConversion  OutDataTypeStr=boolean
  ToBool_Fault : DataTypeConversion  OutDataTypeStr=boolean
  ToBool_GridConnected : DataTypeConversion  OutDataTypeStr=boolean
  Unit Delay8 : UnitDelay  SampleTime=-1  HasFrameUpgradeWarning=on
  Vdc_Input_Delay : UnitDelay  InitialCondition=Vdc_ref  SampleTime=Ts_ems
  Ppv_ems : Outport  OutDataTypeStr=double  PortDimensions=1
  Pdc_ems : Outport  Port=2  OutDataTypeStr=double  PortDimensions=1
  Vabc_load_fast : Outport  Port=3  OutDataTypeStr=double  PortDimensions=3
  Iabc_load_fast : Outport  Port=4  OutDataTypeStr=double  PortDimensions=3
  Pgrid_ems : Outport  Port=5  OutDataTypeStr=double  PortDimensions=1
  Pbat_ems : Outport  Port=6  OutDataTypeStr=double  PortDimensions=1
  Vdc_ems : Outport  Port=7  OutDataTypeStr=double  PortDimensions=1
  Vbat_ems : Outport  Port=8  OutDataTypeStr=double  PortDimensions=1
  SOC_ems : Outport  Port=9  OutDataTypeStr=double  PortDimensions=1
  GridConnected_ems : Outport  Port=10  OutDataTypeStr=boolean  PortDimensions=1
  EMS_enable_ems : Outport  Port=11  OutDataTypeStr=boolean  PortDimensions=1
  Fault_ems : Outport  Port=12  OutDataTypeStr=boolean  PortDimensions=1
  wires:
  RT_Fault/1 -> Fault_ems/1
  ToBool_Fault/1 -> RT_Fault/1
  Fault/1 -> ToBool_Fault/1
  RT_EMS_enable/1 -> EMS_enable_ems/1
  ToBool_EMS_enable/1 -> RT_EMS_enable/1
  EMS_enable/1 -> ToBool_EMS_enable/1
  ToBool_GridConnected/1 -> RT_GridConnected/1
  GridConnected/1 -> ToBool_GridConnected/1
  RT_SOC/1 -> SOC_ems/1
  SOC/1 -> RT_SOC/1
  RT_Vbat/1 -> Vbat_ems/1
  Vdc_Input_Delay/1 -> Vdc_ems/1
  RT_Vdc/1 -> Vdc_Input_Delay/1
  RT_Pbat/1 -> Pbat_ems/1
  Pbat_meas/1 -> Battery_Power_Sign/1
  RT_Pgrid/1 -> Pgrid_ems/1
  Grid_Power_Sign/1 -> RT_Pgrid/1
  Iabc_load/1 -> Iabc_load_fast/1
  Vabc_load/1 -> Vabc_load_fast/1
  RT_Pdc/1 -> Pdc_ems/1
  Pdc/1 -> RT_Pdc/1
  RT_Ppv/1 -> Ppv_ems/1
  Ppv/1 -> RT_Ppv/1
  Battery_Power_Sign/1 -> MA_Pbat/1
  MA_Pbat/1 -> RT_Pbat/1
  Vdc/1 -> MA_Vdc/1
  MA_Vdc/1 -> RT_Vdc/1
  Vbat/1 -> MA_Vbat/1
  MA_Vbat/1 -> RT_Vbat/1
  RT_GridConnected/1 -> Switch9/2, GridConnected_ems/1
  Unit Delay8/1 -> Sum12/1
  Sum12/1 -> Saturation3/1
  Constant41/1 -> Sum12/2
  Saturation3/1 -> Switch9/1
  Constant42/1 -> Switch9/3
  Switch9/1 -> Product/1, Unit Delay8/1  "alpha"
  Pgrid_meas/1 -> Product/2
  Product/1 -> Grid_Power_Sign/1

== matlab function manul_model_stage15_complete_pre_engineering_20260816/MATLAB Function ==
  data: Iref input; Iout output; SOC input; SOC_min input; SOC_max input
function Iout = SOC_Protection(Iref, SOC, SOC_min, SOC_max)

if SOC <= SOC_min
    Iout = min(Iref, 0);   % SOC过低：禁止正电流放电

elseif SOC >= SOC_max
    Iout = max(Iref, 0);   % SOC过高：禁止负电流充电

else
    Iout = Iref;           % 正常SOC：不限制
end

end

== matlab function manul_model_stage15_complete_pre_engineering_20260816/MATLAB Function2 ==
  data: Vdc input; gates output; Vg_ab input; P input; Q input; Pref input; Qref input; Ts input; Lf input; Rf input; omega input; Pbase input; Qbase input; lambda_sw input; previousState input; stateIndex output; Jmin output
function [gates,stateIndex,Jmin] = pvess_mppc_block( ...
    Vdc,Vg_ab,P,Q,Pref,Qref,Ts,Lf,Rf,omega,Pbase,Qbase, ...
    lambda_sw,previousState)
%PVESS_MPPC_BLOCK Code for the grid-connected MATLAB Function block.
% Copy this whole function into a MATLAB Function block, or call it from
% that block. The equations follow the paper's P/Q predictive model.
%
% IMPORTANT SIGN CONVENTION:
% P,Q and the measured current must use one consistent direction.
% SIGN CONVENTION:
% Filter current If is positive from inverter toward grid.
% Positive active power P means power exported from inverter/microgrid
% toward the grid. 
% If the Current Measurement arrow points from
% converter toward grid, multiply that current by -1 before P/Q calculation.

states = [0 0 0; ...
          1 0 0; ...
          1 1 0; ...
          0 1 0; ...
          0 1 1; ...
          0 0 1; ...
          1 0 1; ...
          1 1 1];

Jmin = inf;
stateIndex = 1;
previousState = previousState(:).';
Vg2 = Vg_ab(1)^2 + Vg_ab(2)^2;

for k = 1:8
    s = states(k,:);
    Vi_alpha = (2/3)*Vdc*(s(1)-0.5*s(2)-0.5*s(3));
    Vi_beta  = (sqrt(3)/3)*Vdc*(s(2)-s(3));

    % real/imaginary parts of Vg*conj(Vi).
    realTerm = Vg_ab(1)*Vi_alpha + Vg_ab(2)*Vi_beta;
    imagTerm = Vg_ab(2)*Vi_alpha - Vg_ab(1)*Vi_beta;

    % Paper active/reactive power one-step prediction.
    Ppred = P + Ts*(-Rf/Lf*P - omega*Q ...
        + 3/(2*Lf)*(realTerm - Vg2));
    Qpred = Q + Ts*( omega*P - Rf/Lf*Q ...
        + 3/(2*Lf)*imagTerm);

    Jpq = ((Pref-Ppred)/Pbase)^2 + ((Qref-Qpred)/Qbase)^2;
    Jsw = lambda_sw*sum(abs(s-previousState));
    J = Jpq + Jsw;

    if J < Jmin
        Jmin = J;
        stateIndex = k;
    end
end

s = states(stateIndex,:);
gates = [s(1);1-s(1);s(2);1-s(2);s(3);1-s(3)];
end

== stateflow chart manul_model_stage15_complete_pre_engineering_20260816/EMS_flowchart ==
  settings: updateMethod=DISCRETE  sampleTime=Ts_ems
  note: EMS
  state Junction_meaning [group]
    J0：并网/孤岛判断
    J1：并网SOC判断
    J2：并网功率不足判断
    J3：孤岛功率判断
    J4：孤岛欠功率SOC判断
    J5：孤岛过剩功率SOC判断
    J6：电池电流映射
    J7：唯一终止节点
  state Variable [group]
    frac表示真实SOC在允许SOC的位置
    也就是电池在允许SOC内还能放多少电
    公式为（SOC-10）/（max-min）
    相当于归一化：
    最后一行在限制输出在0-1，避免异常SOC
    使frac大于1或小于0
    loadShed：负载切除指令
    offMPPT：MPPT关闭指令
  note: J0
  note: J1
  note: J3
  note: J5
  note: J2
  note: J4
  note: J6
  (default) -> (junction 28) : {battCmd = 0.0;
      | Ibat_ref = 0.0;
      | ShedReq = false;
      | offMPPTReq = false;
      | Pnet = Ppv - Pac - Pdc;
      | SOC_mid = 0.5 * (SOC_min + SOC_max);
      | frac = (SOC - SOC_min) / (SOC_max - SOC_min);
      | frac = min(max(frac,0.0),1.0);
      | }
  (junction 28) -> (junction 31) [order 2]
  (junction 28) -> (junction 30) [order 1] : [GridConnected > 0.5]
  (junction 31) -> (junction 93) [order 3]
  (junction 31) -> (junction 49) [order 2] : [Pnet >Pnet_dead]
  (junction 30) -> (junction 41) [order 2]
  (junction 31) -> (junction 46) [order 1] : [Pnet < -Pnet_dead]
  (junction 30) -> (junction 34) [order 1] : [SOC < SOC_mid]{battCmd = -1.0;}
  (junction 93) -> (junction 34) : {battCmd = 0.0;}
  (junction 49) -> (junction 34) [order 2] : {battCmd = 0.0;
      | offMPPTReq = true;}
  (junction 49) -> (junction 34) [order 1] : [SOC < SOC_max]{battCmd = -1.0;}
  (junction 41) -> (junction 34) [order 1] : [Pnet < 0.0 ]{battCmd = 0.0;}
  (junction 41) -> (junction 34) [order 2] : {battCmd = 0.0;}
  (junction 46) -> (junction 34) [order 1] : [SOC > SOC_min]{battCmd = 1.0;}
  (junction 46) -> (junction 34) [order 2] : {battCmd = 0.0;
      | ShedReq = true;}
  (junction 34) -> (junction 58) [order 4] : {Ibat_ref = 0.0;}
  (junction 34) -> (junction 58) [order 2] : [battCmd < -0.5&& SOC < SOC_max&& GridConnected <= 0.5]{Ibat_ref = -min(max(Pnet / V_bat_nom, 0.0), Ibat_max);}
  (junction 34) -> (junction 58) [order 3] : [battCmd < -0.5 && SOC < SOC_max && GridConnected > 0.5]{Ibat_ref = -Ibat_max * (1.0 - frac);}
  (junction 34) -> (junction 58) [order 1] : [battCmd > 0.5&& SOC > SOC_min]{Ibat_ref = min(max(-Pnet / V_bat_nom, 0.0), Ibat_max);}
  data: Ppv input; Pac input; Pdc input; SOC input; GridConnected input double; Ibat_ref output double; SOC_max parameter double; SOC_min parameter double; SOC_mid local double size=[1 1]; frac local double size=[1 1]; Pnet local double size=[1 1]; Ibat_max parameter double; battCmd output double; ShedReq output boolean; offMPPTReq output boolean; V_bat_nom parameter double; Pnet_dead constant double =30e3

== stateflow chart manul_model_stage15_complete_pre_engineering_20260816/ProtectionLogic ==
  state LoadShedlogic [parallel]
    settings: executionOrder=1
    state LoadNormal
      entry:
      loadShed = false;
      during:
      loadShed = false;
    state LoadShed
      entry:
      loadShed = true;
      during:
      loadShed = true;
    LoadNormal -> LoadShed : [ShedReq]
    (default) -> LoadNormal
    LoadShed -> LoadNormal : [after(Tshed_hold,sec) && SOC >= SOC_min + dSOC_shed]
  state offMPPTlogic [parallel]
    settings: executionOrder=2
    state MPPTNormal
      entry:
      offMPPT = false;
      during:
      offMPPT = false;
    state offMPPT
      entry:
      offMPPT = true;
      during:
      offMPPT = true;
    MPPTNormal -> offMPPT : [offMPPTReq]
    (default) -> MPPTNormal
    offMPPT -> MPPTNormal : [after(ToffMPPT_hold,sec) && SOC <= SOC_max - dSOC_mppt]
  data: SOC_max parameter double; SOC_min parameter double; ShedReq input; ToffMPPT_hold constant double =0.2; Tshed_hold constant double =0.2; dSOC_mppt constant double =0.02; dSOC_shed constant double =0.02; offMPPTReq input boolean; loadShed output boolean; offMPPT output boolean; SOC input double

== matlab function manul_model_stage15_complete_pre_engineering_20260816/MATLAB Function1 ==
  data: Vdc input; gates output; Vc_ab input; If_ab input; IL_ab input; Vref_ab input; Ad input; Bd input; lambda_sw input; previousState input; stateIndex output; Jmin output
function [gates,stateIndex,Jmin] = pvess_mpvc_block( ...
    Vdc,Vc_ab,If_ab,IL_ab,Vref_ab,Ad,Bd,lambda_sw,previousState)
%PVESS_MPVC_BLOCK Code for the island-mode MATLAB Function block.
% Copy this whole function into a MATLAB Function block, or call it from
% that block. All vector inputs are real 2-by-1 alpha-beta vectors.
%
% Gate order for the SPS Universal Bridge is:
% [A_upper; A_lower; B_upper; B_lower; C_upper; C_lower].

states = [0 0 0; ...
          1 0 0; ...
          1 1 0; ...
          0 1 0; ...
          0 1 1; ...
          0 0 1; ...
          1 0 1; ...
          1 1 1];

Jmin = inf;
stateIndex = 1;
previousState = previousState(:).';

for k = 1:8
    s = states(k,:);

    % Two-level bridge voltage vector in stationary alpha-beta axes.
    Vi_alpha = (2/3)*Vdc*(s(1)-0.5*s(2)-0.5*s(3));
    Vi_beta  = (sqrt(3)/3)*Vdc*(s(2)-s(3));

    % Paper Eq. (11), independently applied to alpha and beta axes.
    xa = Ad*[Vc_ab(1);If_ab(1)] + Bd*[Vi_alpha;IL_ab(1)];
    xb = Ad*[Vc_ab(2);If_ab(2)] + Bd*[Vi_beta; IL_ab(2)];

    voltageScale = max(Vref_ab(1)^2 + Vref_ab(2)^2,1);
    Jv = ((Vref_ab(1)-xa(1))^2 + (Vref_ab(2)-xb(1))^2) ...
        / voltageScale;
    Jsw = lambda_sw*sum(abs(s-previousState));
    J = Jv + Jsw;

    if J < Jmin
        Jmin = J;
        stateIndex = k;
    end
end

s = states(stateIndex,:);
gates = [s(1);1-s(1);s(2);1-s(2);s(3);1-s(3)];
end
